simulink model "lane_detection_hough"  (R2015b)
settings: Solver=VariableStepAuto  StartTime=0.0  StopTime=inf  RelTol=1e-3
undefined symbols (not defined in the file): gray, Rec, SDTV
libraries: visionsinks x3, visionconversions x2, visiontransforms x2, visionfilter x1, visionstatistics x1, dspvision x1, visiontextngfix x1
settings Model: Creator=Monty  LastModifiedBy=Monty

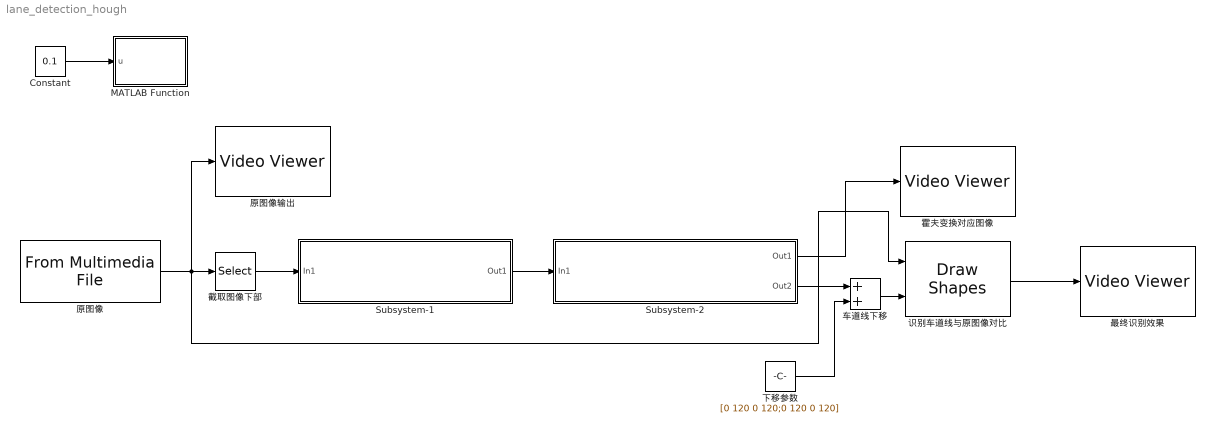
== system lane_detection_hough ==
  Constant : Constant  Value=0.1
  MATLAB Function : MATLAB Function  TreatAsAtomicUnit=on
  Subsystem-1 : Subsystem
      mask Display:
      | disp('图像预处理\n信息1901邱剑楠')
      | port_label('input',1,'视频输入')
      | port_label('output',1,'预处理后图像')
  Subsystem-2 : Subsystem
      mask Display:
      | disp('识别车道线\n信息1901邱剑楠')
      | port_label('input',1,'预处理后的图像')
      | port_label('output',1,'Hough变换图像')
      | port_label('output',2,'车道线')
  下移参数 : Constant  Value=[0 120 0 120;0 120 0 120]
  原图像 : dspvision/From Multimedia File  inputFilename=E:\STUDY\CIRCUIT\Matlab 2015b win64\Matlab 2015b win64\MATLAB\R2015b\toolbox\vision\visiondata\viplanedeparture.avi  loop=on  numPlays=inf  outputStreams=Video only  videoDataType=single  audioDataType=int16  inheritSampleTime=on  userDefinedSampleTime=1/30  noAudioOutput=off  isIntensityVideo=off  fourcc=RGB  colorVideoFormat=One multidimensional signal  outputEOF=off  dataOrg=Column-major  audioFrameSize=1024  computeAudioFrameSize=off  outSamplingMode=Sample based
  原图像输出 : visionsinks/Video Viewer  inputType=Obsolete7b  imagePorts=One multidimensional signal  useColorMap=off  colormapValue=gray(256)  specRange=off  minInputVal=0  maxInputVal=255  FigPos=[485.8 730 409.6 299.2]  AxisZoom=on  trueSizedOnce=off  OpenAtMdlStart=on  DefaultConfigurationName=vipscopes.VideoViewerScopeCfg
  截取图像下部 : Selector  NumberOfDimensions=3  InputPortWidth=3  IndexOptions=Index vector (dialog),Select all,Select all  Indices=[121:240],1,1  OutputSizes=1,1,1
  最终识别效果 : visionsinks/Video Viewer  inputType=Obsolete7b  imagePorts=One multidimensional signal  useColorMap=off  colormapValue=gray(256)  specRange=off  minInputVal=0  maxInputVal=255  FigPos=[940.2 746 409.6 300]  AxisZoom=on  trueSizedOnce=off  OpenAtMdlStart=on  DefaultConfigurationName=vipscopes.VideoViewerScopeCfg
  识别车道线与原图像对比 : visiontextngfix/Draw Shapes  shape=Lines  fill=off  lineWidth=2  fillClrSource=Specify via dialog  display=User-specified value  intensity=200  color=[1 1 0]  opacity=0.6  viewport=Entire image  antialiasing=off  inType=Obsolete  imagePorts=One multidimensional signal  prodOutputMode=Binary point scaling  prodOutputWordLength=32  prodOutputFracLength=14  memoryMode=Specify word length  memoryWordLength=16  memoryFracLength=14  roundingMode=Floor  overflowMode=off
  车道线下移 : Sum
  霍夫变换对应图像 : visionsinks/Video Viewer  inputType=Obsolete7b  imagePorts=One multidimensional signal  useColorMap=off  colormapValue=gray(256)  specRange=off  minInputVal=0  maxInputVal=255  FigPos=[61 725.2 409.6 300]  AxisZoom=on  trueSizedOnce=off  OpenAtMdlStart=on  DefaultConfigurationName=vipscopes.VideoViewerScopeCfg
  wires:
  原图像/1 -> 原图像输出/1, 识别车道线与原图像对比/1, 截取图像下部/1
  Constant/1 -> MATLAB Function/1(u)
  截取图像下部/1 -> Subsystem-1/1(In1)
  Subsystem-1/1(Out1) -> Subsystem-2/1(In1)
  Subsystem-2/1(Out1) -> 霍夫变换对应图像/1
  识别车道线与原图像对比/1 -> 最终识别效果/1
  车道线下移/1 -> 识别车道线与原图像对比/2
  下移参数/1 -> 车道线下移/2
  Subsystem-2/2(Out2) -> 车道线下移/1

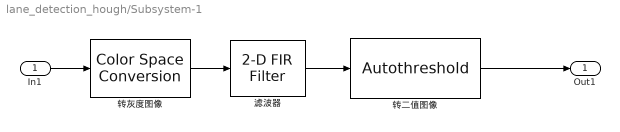
== system lane_detection_hough/Subsystem-1 ==
  In1 : Inport
  滤波器 : visionfilter/2-D FIR Filter  separable=off  filtSrc=Specify via dialog  filterMtrx=[-5 0 5]  verticalFilter=[4 0]  horizontalFilter=[4 0]  outSize=Same as input port I  padType=Symmetric  padSrc=Specify via dialog  padVal=0  method=Convolution  firstCoeffMode=Specify word length  firstCoeffWordLength=16  firstCoeffFracLength=14  firstCoeffSignedness=Signed  firstCoeffDataTypeStr=fixdt(1,16)  firstCoeffLastDataTypeStr=fixdt(1,16)  firstCoeffMin=[]  firstCoeffMax=[]  outputSignedness=Auto  outputMin=[]  outputMax=[]  accumDataTypeStr=Inherit: Same as product output  accumLastDataTypeStr=Inherit: Same as product output  prodOutputMode=Binary point scaling  prodOutputWordLength=32  prodOutputFracLength=10  prodOutputDataTypeStr=fixdt([],32,10)  prodOutputLastDataTypeStr=fixdt([],32,10)  roundingMode=Floor  overflowMode=off
  转二值图像 : visionconversions/Autothreshold  operator=>  threshOut=off  effMetricOut=off  userDefinedRange=off  umin=0  umax=255  outOfRngOpt=Warn and saturate  scaleThreshold=off  scaleFactor=1  P1Mode=Specify word length  P1WordLength=32  P1FracLength=30  P2Mode=Specify word length  P2WordLength=32  P2FracLength=22  P3Mode=Specify word length  P3WordLength=32  P3FracLength=14  P4Mode=Binary point scaling  P4WordLength=32  P4FracLength=15  Q1Mode=Specify word length  Q1WordLength=32  Q1FracLength=16  EMMode=Specify word length  EMWordLength=16  EMFracLength=14  roundingMode=Floor  overflowMode=off
  "转灰度图像 " : visionconversions/Color Space  Conversion  conversion=Obsolete  conversionActive=R'G'B' to intensity  wp_str=D65  rec=Rec. 601 (SDTV)  sys=1125/60/2:1  imagePorts=One multidimensional signal
  Out1 : Outport
  wires:
  转二值图像/1 -> Out1/1
  In1/1 -> "转灰度图像 "/1
  滤波器/1 -> 转二值图像/1
  "转灰度图像 "/1 -> 滤波器/1

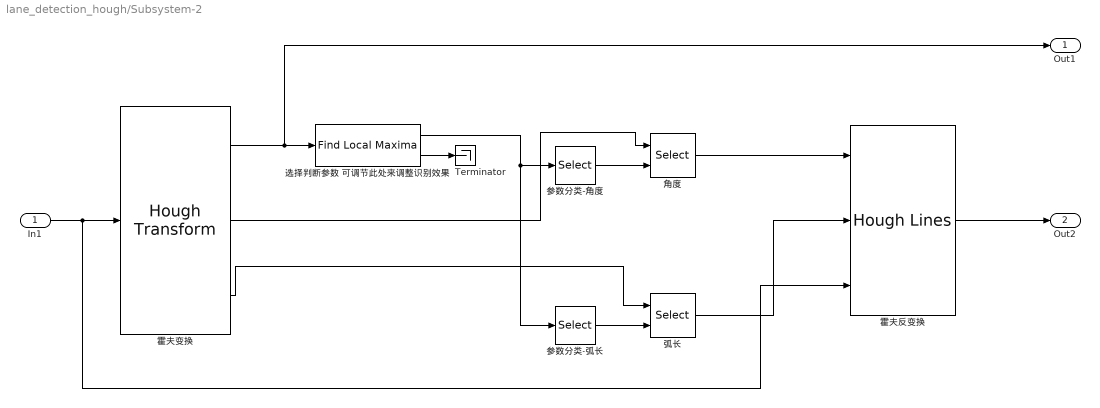
== system lane_detection_hough/Subsystem-2 ==
  In1 : Inport
  Terminator : Terminator
  参数分类-弧长 : Selector  NumberOfDimensions=2  InputPortWidth=3  IndexOptions=Select all,Index vector (dialog)  Indices=[1 3],2  OutputSizes=1,1
  参数分类-角度 : Selector  NumberOfDimensions=2  InputPortWidth=3  IndexOptions=Select all,Index vector (dialog)  Indices=[1 3],1  OutputSizes=1,1
  弧长 : Selector  IndexMode=Zero-based  IndexOptions=Index vector (port)  Indices=[1 3]  OutputSizes=1
  角度 : Selector  IndexMode=Zero-based  IndexOptions=Index vector (port)  Indices=[1 3]  OutputSizes=1
  选择判断参数 可调节此处来调整识别效果 : visionstatistics/Find Local Maxima  num_peaks=2  nhood_size=[235 57]  src_thresh=Obsolete9b  src_thresh_inuse=Specify via dialog  threshold=10  inputIsHough=off  dt_peak=uint32  isOutVarDim=off  dt_count=uint32
  霍夫反变换 : visiontransforms/Hough Lines  sineCompMethod=Trigonometric function  thetaRes=pi/180  firstCoeffMode=Specify word length  firstCoeffWordLength=16  firstCoeffFracLength=15  prodOutputMode=Binary point scaling  prodOutputWordLength=32  prodOutputFracLength=16  roundingMode=Nearest  overflowMode=on
  霍夫变换 : visiontransforms/Hough Transform  theta_res=pi/180  rho_res=1  out_theta_rho=on  outdtmode=double  firstCoeffMode=Binary point scaling  firstCoeffWordLength=16  firstCoeffFracLength=14  secondCoeffMode=Binary point scaling  secondCoeffWordLength=32  secondCoeffFracLength=16  outputMode=Binary point scaling  outputWordLength=16  outputFracLength=0  accumMode=Binary point scaling  accumWordLength=32  accumFracLength=20  prodOutputMode=Binary point scaling  prodOutputWordLength=32  prodOutputFracLength=20  memoryMode=Binary point scaling  memoryWordLength=32  memoryFracLength=16  roundingMode=Nearest  overflowMode=on
  Out1 : Outport
  Out2 : Outport  Port=2
  wires:
  霍夫变换/3 -> 弧长/1
  参数分类-弧长/1 -> 弧长/2
  弧长/1 -> 霍夫反变换/2
  选择判断参数 可调节此处来调整识别效果/1 -> 参数分类-弧长/1, 参数分类-角度/1
  参数分类-角度/1 -> 角度/2
  霍夫变换/2 -> 角度/1
  角度/1 -> 霍夫反变换/1
  In1/1 -> 霍夫反变换/3, 霍夫变换/1
  霍夫变换/1 -> Out1/1, 选择判断参数 可调节此处来调整识别效果/1
  霍夫反变换/1 -> Out2/1
  选择判断参数 可调节此处来调整识别效果/2 -> Terminator/1

== matlab function lane_detection_hough/MATLAB Function ==
  data: u input
function fcn(u)
%#codegen

pause(u);
